simulink model "vienna"  (R2021a)
settings: Solver=VariableStepAuto  StartTime=0.0  StopTime=10.0  RelTol=1e-3
libraries: spsDiodeLib x6, spsMosfetLib x6, pid_lib x4, spsSeriesRLCBranchLib x3, spsVoltageMeasurementLib x3, powerlib_extras x3, simulink x1, spsThreePhaseSeriesRLCBranchLib x1, spsThreePhaseVIMeasurementLib x1, spsThreePhaseSourceLib x1, spsPLL3phLib x1, spspowerguiLib x1
settings Model: Creator=DSH  LastModifiedBy=DSH

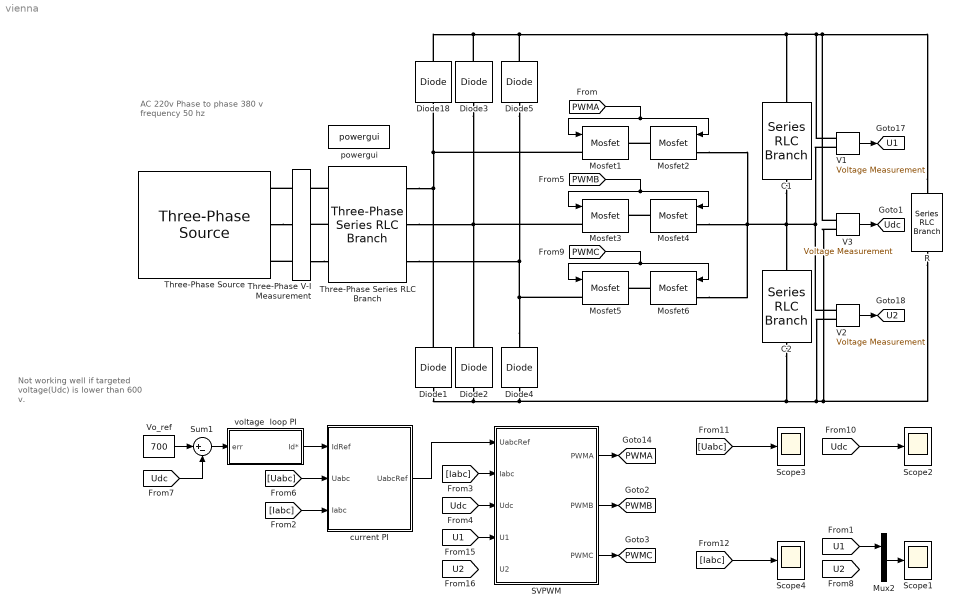
== system vienna ==
  note: AC 220v
      | Phase to phase 380 v
      | frequency 50 hz
  note: Not working well if
      | targeted voltage(Udc)
      | is lower than 600 v.
  C1 : spsSeriesRLCBranchLib/Series RLC Branch  LConnTagsString=__new0  RConnTagsString=__new0  BranchType=C  Resistance=0.1  Inductance=1e-3  SetiL0=off  InitialCurrent=0  Capacitance=1087e-6  Setx0=on  InitialVoltage=0  Measurements=None
  C2 : spsSeriesRLCBranchLib/Series RLC Branch  LConnTagsString=__new0  RConnTagsString=__new0  BranchType=C  Resistance=0.1  Inductance=1e-3  SetiL0=off  InitialCurrent=0  Capacitance=1087e-6  Setx0=on  InitialVoltage=0  Measurements=None
  Diode{1..5,18} (6 alike) : spsDiodeLib/Diode  Ron=0.001  Lon=0  Vf=0.8  IC=0  UseSnubber=off  Rs=500  Cs=250e-9  Measurements=off
  Mosfet{1..6} (6 alike) : spsMosfetLib/Mosfet  Ron=0.1  Lon=0  Rd=0.01  Vfd=0  IC=0  Rs=1e5  Cs=inf  Measurements=off
  Mux2 : Mux  Inputs=2
  R : spsSeriesRLCBranchLib/Series RLC Branch  LConnTagsString=__new0  RConnTagsString=__new0  BranchType=R  Resistance=10  Inductance=1e-3  SetiL0=off  InitialCurrent=0  Capacitance=100e-6  Setx0=off  InitialVoltage=0  Measurements=None
  SVPWM : Subsystem
  Scope{1..4} (4 alike) : Scope
  Sum1 : Sum  Inputs=|+-  SampleTime=1e-5
  Three-Phase Series RLC Branch : spsThreePhaseSeriesRLCBranchLib/Three-Phase Series RLC Branch  LConnTagsString=A|B|C  RConnTagsString=A|B|C  BranchType=L  Resistance=0.05  Inductance=0.406e-3  Capacitance=1e-6  Measurements=None
  Three-Phase V-I Measurement : spsThreePhaseVIMeasurementLib/Three-Phase V-I Measurement  VoltageMeasurement=phase-to-ground  SetLabelV=on  LabelV=Uabc  Vpu=off  VpuLL=off  CurrentMeasurement=yes  SetLabelI=on  LabelI=Iabc  Ipu=off  Pbase=100e6  Vbase=500e3  OutputType=Complex  PhasorSimulation=off  PSBequivalent=0
  Three-Phase Source : spsThreePhaseSourceLib/Three-Phase Source  InternalConnection=Yg  VoltagePhases=off  Voltage=380  PhaseAngle=0  Voltage_phases=[25e3 25e3 25e3]/sqrt(3)  PhaseAngles_phases=[0 -120 +120]  Frequency=50  NonIdealSource=on  SpecifyImpedance=off  Resistance=0.000001  Inductance=0  ShortCircuitLevel=100e6  BaseVoltage=25e3  XRratio=7  BusType=swing  Pref=0  Qref=0  Prefabc=[10e3, 10e3, 10e3]  Qrefabc=[0, 0, 0]  Qmin=-inf  Qmax=inf
  V1 : spsVoltageMeasurementLib/Voltage Measurement  PhasorSimulation=off  OutputType=Complex  PSBequivalent=0
  V2 : spsVoltageMeasurementLib/Voltage Measurement  PhasorSimulation=off  OutputType=Complex  PSBequivalent=0
  V3 : spsVoltageMeasurementLib/Voltage Measurement  PhasorSimulation=off  OutputType=Complex  PSBequivalent=0
  Vo_ref : Constant  Value=700
  current PI : Subsystem
  powergui : spspowerguiLib/powergui  Priority=1  SimulationMode=Discrete  SampleTime=1e-7  frequency=60  Iterations=50  frequencyindice=0  Pbase=100e6  ErrMax=1e-4  UnitsV=kV  UnitsW=MW  buscounter=0  FunctionMessages=off  echomessages=off  EnableUseOfTLC=off  CurrentSourceSwitches=off  DisableSnubberDevices=off  DisableRonSwitches=off  DisableVfSwitches=off  DisplayEquations=off  AutomaticDiscreteSolvers=off  SolverType=Tustin  Interpol=off  ExternalGateDelay=off  methode=off  Ts=0  x0status=blocks  SPID=off  SwTol=0  HookPort=off  NonlinearTolerance=1e-4  nMaxIteration=100  ContinueOnMaxIteration=off  RestoreLinks=warning  ResistiveCurrentMeasurement=off  Frange=[0:2:500]  Ylog=off  Xlog=on  ShowGrid=off  save=off  variable=ZData  structure=output  ZoomFFT=off  StartTime=0.1  cycles=20  DisplayStyle=1  fundamental=400  FreqAxis=off  MaxFrequency=20000  frequencyindicesteady=1  RmsSteady=1  display=off
  voltage  loop PI : Subsystem
      mask Display: disp('PI')
  tag scope: PWMA=global, PWMB=global, PWMC=global, U1=global, U2=global, Udc=global
  wires:
  [Iabc] -> Scope4/1
  [Iabc] -> SVPWM/2(Iabc)
  [Iabc] -> current PI/3(Iabc)
  Sum1/1 -> voltage  loop PI/1(err)
  [Uabc] -> Scope3/1
  [U1] -> Mux2/1
  [U1] -> SVPWM/4(U1)
  SVPWM/1(PWMA) -> [PWMA]
  Mux2/1 -> Scope1/1
  [Udc] -> Scope2/1
  V3/1 -> [Udc]
  [PWMB] -> Mosfet4/1, Mosfet3/1
  [PWMC] -> Mosfet5/1, Mosfet6/1
  [PWMA] -> Mosfet1/1, Mosfet2/1
  voltage  loop PI/1(Id*) -> current PI/1(IdRef)
  [Udc] -> SVPWM/3(Udc)
  [Uabc] -> current PI/2(Uabc)
  V2/1 -> [U2]
  Vo_ref/1 -> Sum1/1
  SVPWM/2(PWMB) -> [PWMB]
  [Udc] -> Sum1/2
  SVPWM/3(PWMC) -> [PWMC]
  V1/1 -> [U1]
  current PI/1(UabcRef) -> SVPWM/1(UabcRef)
  connections:
  R/LConn1 -- Diode5/RConn1 -- Diode18/RConn1 -- Diode3/RConn1 -- C1/LConn1 -- V1/LConn1 -- V3/LConn1
  Three-Phase Series RLC Branch/RConn1 -- Diode1/RConn1 -- Mosfet1/LConn1 -- Diode18/LConn1
  Diode4/LConn1 -- Diode1/LConn1 -- Diode2/LConn1 -- C2/RConn1 -- V2/LConn2 -- R/RConn1 -- V3/LConn2
  Three-Phase Series RLC Branch/RConn2 -- Diode3/LConn1 -- Mosfet3/LConn1 -- Diode2/RConn1
  V1/LConn2 -- Mosfet2/LConn1 -- Mosfet6/LConn1 -- Mosfet4/LConn1 -- C2/LConn1 -- C1/RConn1 -- V2/LConn1
  Diode4/RConn1 -- Diode5/LConn1 -- Three-Phase Series RLC Branch/RConn3 -- Mosfet5/LConn1
  Three-Phase Series RLC Branch/LConn1 -- Three-Phase V-I Measurement/RConn1
  Mosfet4/RConn1 -- Mosfet3/RConn1
  Mosfet6/RConn1 -- Mosfet5/RConn1
  Mosfet2/RConn1 -- Mosfet1/RConn1
  Three-Phase V-I Measurement/LConn1 -- Three-Phase Source/RConn1
  Three-Phase V-I Measurement/RConn3 -- Three-Phase Series RLC Branch/LConn3
  Three-Phase Series RLC Branch/LConn2 -- Three-Phase V-I Measurement/RConn2
  Three-Phase Source/RConn2 -- Three-Phase V-I Measurement/LConn2
  Three-Phase V-I Measurement/LConn3 -- Three-Phase Source/RConn3

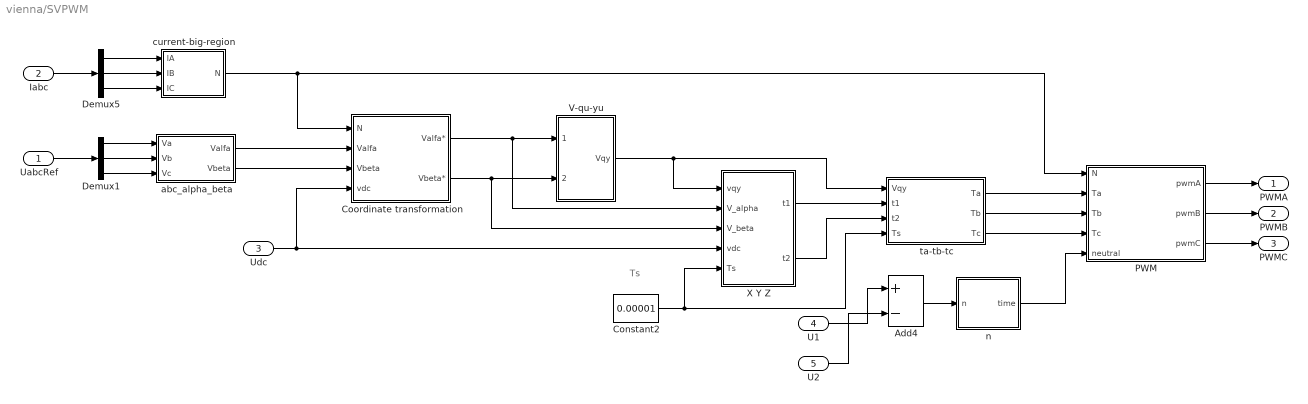
== system vienna/SVPWM ==
  note: Ts
  UabcRef : Inport
  Iabc : Inport  Port=2
  Udc : Inport  Port=3
  U1 : Inport  Port=4
  U2 : Inport  Port=5
  Add4 : Sum  Inputs=+-
  Constant2 : Constant  Value=0.00001
  Coordinate transformation : Subsystem
  Demux1 : Demux  Outputs=3
  Demux5 : Demux  Outputs=3
  PWM : Subsystem
  "V-qu-yu " : Subsystem
  X Y Z : Subsystem
  abc_alpha_beta : Subsystem
  current-big-region : Subsystem
  n : Subsystem
  ta-tb-tc : Subsystem
  PWMA : Outport
  PWMB : Outport  Port=2
  PWMC : Outport  Port=3
  wires:
  Demux1/3 -> abc_alpha_beta/3(Vc)
  Demux1/2 -> abc_alpha_beta/2(Vb)
  Demux1/1 -> abc_alpha_beta/1(Va)
  Demux5/2 -> current-big-region/2(IB)
  Demux5/1 -> current-big-region/1(IA)
  Demux5/3 -> current-big-region/3("IC ")
  abc_alpha_beta/2(Vbeta) -> Coordinate transformation/3("Vbeta ")
  Udc/1 -> X Y Z/4(vdc), Coordinate transformation/4(vdc)
  Coordinate transformation/2(Vbeta*) -> "V-qu-yu "/2(Vbeta*), X Y Z/3(V_beta)
  Coordinate transformation/1(Valfa*) -> "V-qu-yu "/1(Valfa*), X Y Z/2(V_alpha)
  Constant2/1 -> X Y Z/5(Ts), ta-tb-tc/4(Ts)
  X Y Z/1(t1) -> ta-tb-tc/2(t1)
  X Y Z/2(t2) -> ta-tb-tc/3(t2)
  ta-tb-tc/2(Tb) -> PWM/3(Tb)
  ta-tb-tc/3(Tc) -> PWM/4(Tc)
  current-big-region/1("N ") -> Coordinate transformation/1(N), PWM/1(N)
  "V-qu-yu "/1("Vqy ") -> ta-tb-tc/1(Vqy), X Y Z/1(vqy)
  ta-tb-tc/1(Ta) -> PWM/2(Ta)
  abc_alpha_beta/1(Valfa) -> Coordinate transformation/2(Valfa)
  Iabc/1 -> Demux5/1
  UabcRef/1 -> Demux1/1
  n/1(time) -> PWM/5(neutral)
  Add4/1 -> n/1(n)
  U1/1 -> Add4/1
  U2/1 -> Add4/2
  PWM/1(pwmA) -> PWMA/1
  PWM/2(pwmB) -> PWMB/1
  PWM/3(pwmC) -> PWMC/1

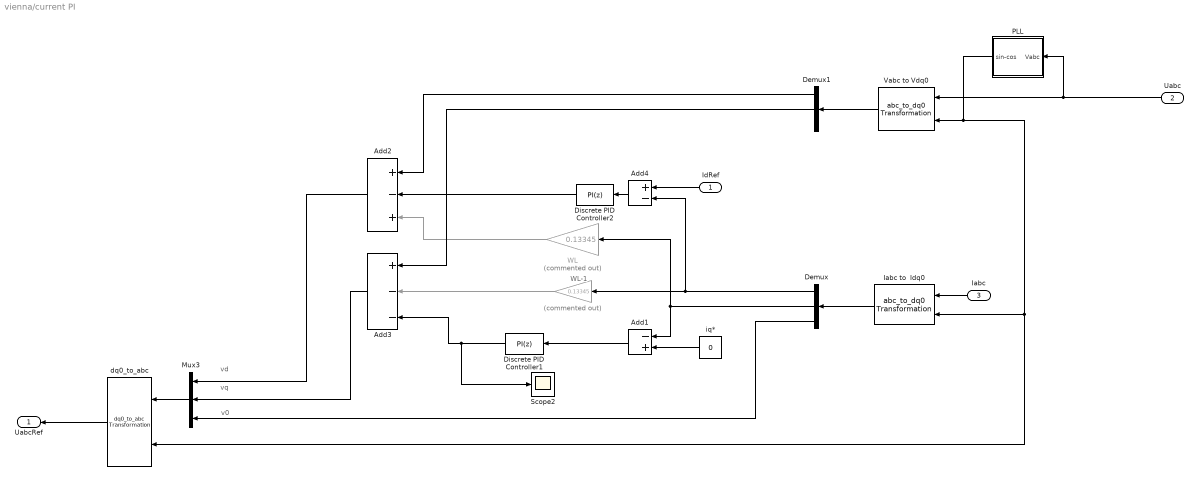
== system vienna/current PI ==
  note: v0
  note: vq
  note: vd
  note: WL-1
  IdRef : Inport
  Uabc : Inport  Port=2
  Iabc : Inport  Port=3
  " " : Gain  Commented=on  Gain=0.13345
  " WL" : Gain  Commented=on  Gain=0.13345
  Add1 : Sum  Inputs=-+
  Add2 : Sum  Inputs=+-+
  Add3 : Sum  Inputs=+--
  Add4 : Sum  Inputs=+-
  Demux : Demux  Outputs=3
  Demux1 : Demux  Outputs=3
  Discrete PID Controller1 : pid_lib/PID Controller  Controller=PI  Form=Parallel  TimeDomain=Discrete-time  UseExternalTs=off  SampleTime=1e-5  IntegratorMethod=Forward Euler  FilterMethod=Forward Euler  ControllerParametersSource=internal  P=0.1  I=100  D=0  UseFilter=on  N=100  TunerSelectOption=Transfer Function Based (PID Tuner App)  InitialConditionSource=internal  InitialConditionForIntegrator=0  InitialConditionForFilter=0  DifferentiatorICPrevScaledInput=0  ExternalReset=none  TrackingMode=off  Kt=1  LimitOutput=on  SatLimitsSource=internal  UpperSaturationLimit=600  LowerSaturationLimit=-600  LinearizeAsGain=off  AntiWindupMode=none  Kb=1  POutMin=[]  POutMax=[]  IOutMin=[]  IOutMax=[]  DOutMin=[]  DOutMax=[]  NOutMin=[]  NOutMax=[]  SumOutMin=[]  SumOutMax=[]  SaturationOutMin=[]  SaturationOutMax=[]  PParamMin=[]  PParamMax=[]  IParamMin=[]  IParamMax=[]  DParamMin=[]  DParamMax=[]  NParamMin=[]  NParamMax=[]  KbParamMin=[]  KbParamMax=[]  KtParamMin=[]  KtParamMax=[]  KbOutMin=[]  KbOutMax=[]  KtOutMin=[]  KtOutMax=[]  IntegratorOutMin=[]  IntegratorOutMax=[]  FilterOutMin=[]  FilterOutMax=[]  SumI1OutMin=[]  SumI1OutMax=[]  SumI2OutMin=[]  SumI2OutMax=[]  SumI3OutMin=[]  SumI3OutMax=[]  SumI4OutMin=[]  SumI4OutMax=[]  SumDOutMin=[]  SumDOutMax=[]  DifferentiatorOutMin=[]  DifferentiatorOutMax=[]  FilterDiffOutCoefMin=[]  FilterDiffOutCoefMax=[]  ReciprocalOutMin=[]  ReciprocalOutMax=[]  SumDenOutMin=[]  SumDenOutMax=[]  SumNumOutMin=[]  SumNumOutMax=[]  DivideOutMin=[]  DivideOutMax=[]  UdiffTsProdOutMin=[]  UdiffTsProdOutMax=[]  NTsProdOutMin=[]  NTsProdOutMax=[]  UintegralTsProdOutMin=[]  UintegralTsProdOutMax=[]  UngainTsProdOutMin=[]  UngainTsProdOutMax=[]  IntegratorContinuousStateAttributes=''  IntegratorStateMustResolveToSignalObject=off  IntegratorRTWStateStorageClass=Auto  FilterContinuousStateAttributes=''  FilterStateMustResolveToSignalObject=off  FilterRTWStateStorageClass=Auto  ParallelPVariant=InternalParameters  IdealPVariant=Disabled  IVariant=InternalParameters  DVariant=Disabled  IntegratorVariant=Discrete  SatVariant=Enabled  AWVariant=Passthrough  PCopyVariant=Disabled  TRVariant=Disabled  FdbkBlocksVariant=Forward  IdealPFdbkVariant=Disabled  SatFdbkVariant=Disabled  DerivativeFilterVariant=Disabled  NVariant=Disabled  NCopyVariant=Disabled_SignalSpec  FilterICVariant=Disabled  IntegratorICVariant=InternalICs  ExternalResetVariant=Disabled  TRSumVariant=Passthrough  SumFdbkVariant=Disabled  SumVariant=Sum_PI  TsampFilterVariant=InternalTs  TsampNgainVariant=Passthrough  TsampIntegralVariant=Passthrough  ExternalSaturationOutDataTypeStr=Inherit: Same as second input
  Discrete PID Controller2 : pid_lib/PID Controller  Controller=PI  Form=Parallel  TimeDomain=Discrete-time  UseExternalTs=off  SampleTime=1e-5  IntegratorMethod=Forward Euler  FilterMethod=Forward Euler  ControllerParametersSource=internal  P=0.1  I=100  D=0  UseFilter=on  N=100  TunerSelectOption=Transfer Function Based (PID Tuner App)  InitialConditionSource=internal  InitialConditionForIntegrator=0  InitialConditionForFilter=0  DifferentiatorICPrevScaledInput=0  ExternalReset=none  TrackingMode=off  Kt=1  LimitOutput=on  SatLimitsSource=internal  UpperSaturationLimit=600  LowerSaturationLimit=-600  LinearizeAsGain=off  AntiWindupMode=none  Kb=1  POutMin=[]  POutMax=[]  IOutMin=[]  IOutMax=[]  DOutMin=[]  DOutMax=[]  NOutMin=[]  NOutMax=[]  SumOutMin=[]  SumOutMax=[]  SaturationOutMin=[]  SaturationOutMax=[]  PParamMin=[]  PParamMax=[]  IParamMin=[]  IParamMax=[]  DParamMin=[]  DParamMax=[]  NParamMin=[]  NParamMax=[]  KbParamMin=[]  KbParamMax=[]  KtParamMin=[]  KtParamMax=[]  KbOutMin=[]  KbOutMax=[]  KtOutMin=[]  KtOutMax=[]  IntegratorOutMin=[]  IntegratorOutMax=[]  FilterOutMin=[]  FilterOutMax=[]  SumI1OutMin=[]  SumI1OutMax=[]  SumI2OutMin=[]  SumI2OutMax=[]  SumI3OutMin=[]  SumI3OutMax=[]  SumI4OutMin=[]  SumI4OutMax=[]  SumDOutMin=[]  SumDOutMax=[]  DifferentiatorOutMin=[]  DifferentiatorOutMax=[]  FilterDiffOutCoefMin=[]  FilterDiffOutCoefMax=[]  ReciprocalOutMin=[]  ReciprocalOutMax=[]  SumDenOutMin=[]  SumDenOutMax=[]  SumNumOutMin=[]  SumNumOutMax=[]  DivideOutMin=[]  DivideOutMax=[]  UdiffTsProdOutMin=[]  UdiffTsProdOutMax=[]  NTsProdOutMin=[]  NTsProdOutMax=[]  UintegralTsProdOutMin=[]  UintegralTsProdOutMax=[]  UngainTsProdOutMin=[]  UngainTsProdOutMax=[]  IntegratorContinuousStateAttributes=''  IntegratorStateMustResolveToSignalObject=off  IntegratorRTWStateStorageClass=Auto  FilterContinuousStateAttributes=''  FilterStateMustResolveToSignalObject=off  FilterRTWStateStorageClass=Auto  ParallelPVariant=InternalParameters  IdealPVariant=Disabled  IVariant=InternalParameters  DVariant=Disabled  IntegratorVariant=Discrete  SatVariant=Enabled  AWVariant=Passthrough  PCopyVariant=Disabled  TRVariant=Disabled  FdbkBlocksVariant=Forward  IdealPFdbkVariant=Disabled  SatFdbkVariant=Disabled  DerivativeFilterVariant=Disabled  NVariant=Disabled  NCopyVariant=Disabled_SignalSpec  FilterICVariant=Disabled  IntegratorICVariant=InternalICs  ExternalResetVariant=Disabled  TRSumVariant=Passthrough  SumFdbkVariant=Disabled  SumVariant=Sum_PI  TsampFilterVariant=InternalTs  TsampNgainVariant=Passthrough  TsampIntegralVariant=Passthrough  ExternalSaturationOutDataTypeStr=Inherit: Same as second input
  Iabc to  Idq0 : powerlib_extras/Measurements/abc_to_dq0 Transformation
      settings: SourceProductBaseCode=PS
  Mux3 : Mux  Inputs=3
  PLL : Subsystem
  Scope2 : Scope
  Vabc to Vdq0 : powerlib_extras/Measurements/abc_to_dq0 Transformation
      settings: SourceProductBaseCode=PS
  dq0_to_abc : powerlib_extras/Measurements/dq0_to_abc Transformation
      settings: SourceProductBaseCode=PS
  iq* : Constant  Value=0
  UabcRef : Outport
  wires:
  " WL"/1 -> Add2/3
  Discrete PID Controller2/1 -> Add2/2
  Demux1/1 -> Add2/1
  Vabc to Vdq0/1 -> Demux1/1
  Uabc/1 -> Vabc to Vdq0/1, PLL/1(Vabc)
  Add3/1 -> Mux3/2
  Add2/1 -> Mux3/1
  Mux3/1 -> dq0_to_abc/1
  Demux/1 -> Add4/2, " "/1
  Demux/3 -> Mux3/3
  dq0_to_abc/1 -> UabcRef/1
  Iabc/1 -> Iabc to  Idq0/1
  Add1/1 -> Discrete PID Controller1/1
  Iabc to  Idq0/1 -> Demux/1
  IdRef/1 -> Add4/1
  Discrete PID Controller1/1 -> Scope2/1, Add3/3
  Demux1/2 -> Add3/1
  " "/1 -> Add3/2
  PLL/1(sin-cos) -> Vabc to Vdq0/2, dq0_to_abc/2, Iabc to  Idq0/2
  Demux/2 -> " WL"/1, Add1/1
  iq*/1 -> Add1/2
  Add4/1 -> Discrete PID Controller2/1

== system vienna/voltage  loop PI ==
  err : Inport
  Discrete PID Controller : pid_lib/PID Controller  Controller=PI  Form=Parallel  TimeDomain=Discrete-time  UseExternalTs=off  SampleTime=1e-5  IntegratorMethod=Forward Euler  FilterMethod=Forward Euler  ControllerParametersSource=internal  P=0.5  I=100  D=0  UseFilter=on  N=100  TunerSelectOption=Transfer Function Based (PID Tuner App)  InitialConditionSource=internal  InitialConditionForIntegrator=0  InitialConditionForFilter=0  DifferentiatorICPrevScaledInput=0  ExternalReset=none  TrackingMode=off  Kt=1  LimitOutput=on  SatLimitsSource=internal  UpperSaturationLimit=150  LowerSaturationLimit=0  LinearizeAsGain=off  AntiWindupMode=none  Kb=1  POutMin=[]  POutMax=[]  IOutMin=[]  IOutMax=[]  DOutMin=[]  DOutMax=[]  NOutMin=[]  NOutMax=[]  SumOutMin=[]  SumOutMax=[]  SaturationOutMin=[]  SaturationOutMax=[]  PParamMin=[]  PParamMax=[]  IParamMin=[]  IParamMax=[]  DParamMin=[]  DParamMax=[]  NParamMin=[]  NParamMax=[]  KbParamMin=[]  KbParamMax=[]  KtParamMin=[]  KtParamMax=[]  KbOutMin=[]  KbOutMax=[]  KtOutMin=[]  KtOutMax=[]  IntegratorOutMin=[]  IntegratorOutMax=[]  FilterOutMin=[]  FilterOutMax=[]  SumI1OutMin=[]  SumI1OutMax=[]  SumI2OutMin=[]  SumI2OutMax=[]  SumI3OutMin=[]  SumI3OutMax=[]  SumI4OutMin=[]  SumI4OutMax=[]  SumDOutMin=[]  SumDOutMax=[]  DifferentiatorOutMin=[]  DifferentiatorOutMax=[]  FilterDiffOutCoefMin=[]  FilterDiffOutCoefMax=[]  ReciprocalOutMin=[]  ReciprocalOutMax=[]  SumDenOutMin=[]  SumDenOutMax=[]  SumNumOutMin=[]  SumNumOutMax=[]  DivideOutMin=[]  DivideOutMax=[]  UdiffTsProdOutMin=[]  UdiffTsProdOutMax=[]  NTsProdOutMin=[]  NTsProdOutMax=[]  UintegralTsProdOutMin=[]  UintegralTsProdOutMax=[]  UngainTsProdOutMin=[]  UngainTsProdOutMax=[]  IntegratorContinuousStateAttributes=''  IntegratorStateMustResolveToSignalObject=off  IntegratorRTWStateStorageClass=Auto  FilterContinuousStateAttributes=''  FilterStateMustResolveToSignalObject=off  FilterRTWStateStorageClass=Auto  ParallelPVariant=InternalParameters  IdealPVariant=Disabled  IVariant=InternalParameters  DVariant=Disabled  IntegratorVariant=Discrete  SatVariant=Enabled  AWVariant=Passthrough  PCopyVariant=Disabled  TRVariant=Disabled  FdbkBlocksVariant=Forward  IdealPFdbkVariant=Disabled  SatFdbkVariant=Disabled  DerivativeFilterVariant=Disabled  NVariant=Disabled  NCopyVariant=Disabled_SignalSpec  FilterICVariant=Disabled  IntegratorICVariant=InternalICs  ExternalResetVariant=Disabled  TRSumVariant=Passthrough  SumFdbkVariant=Disabled  SumVariant=Sum_PI  TsampFilterVariant=InternalTs  TsampNgainVariant=Passthrough  TsampIntegralVariant=Passthrough  ExternalSaturationOutDataTypeStr=Inherit: Same as second input
  Id* : Outport
  wires:
  err/1 -> Discrete PID Controller/1
  Discrete PID Controller/1 -> Id*/1

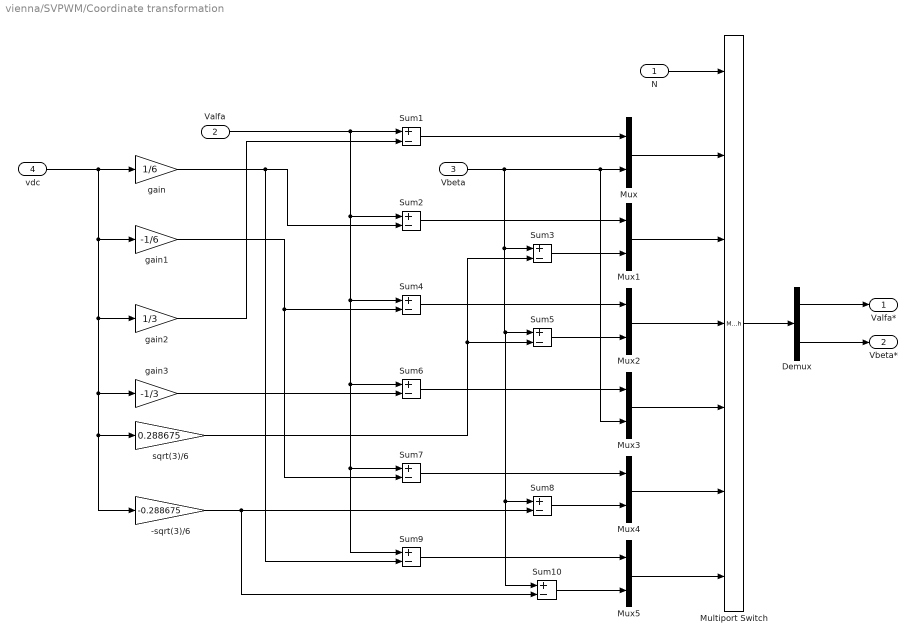
== system vienna/SVPWM/Coordinate transformation ==
  N : Inport
  Valfa : Inport  Port=2
  "Vbeta " : Inport  Port=3
  vdc : Inport  Port=4
  -sqrt(3)/6 : Gain  Gain=-0.288675
  Demux : Demux  Outputs=2
  Multiport Switch : MultiPortSwitch  Inputs=6
  Mux{,1..5} (6 alike) : Mux  Inputs=2
  Sum{1..10} (10 alike) : Sum  Inputs=+-  SaturateOnIntegerOverflow=on
  gain : Gain  Gain=1/6
  gain1 : Gain  Gain=-1/6
  gain2 : Gain  Gain=1/3
  gain3 : Gain  Gain=-1/3
  sqrt(3)/6 : Gain  Gain=0.288675
  Valfa* : Outport
  Vbeta* : Outport  Port=2
  wires:
  Multiport Switch/1 -> Demux/1
  Demux/1 -> Valfa*/1
  Demux/2 -> Vbeta*/1
  N/1 -> Multiport Switch/1
  Mux/1 -> Multiport Switch/2
  Mux1/1 -> Multiport Switch/3
  Mux2/1 -> Multiport Switch/4
  Mux3/1 -> Multiport Switch/5
  Mux4/1 -> Multiport Switch/6
  Mux5/1 -> Multiport Switch/7
  vdc/1 -> gain/1, gain1/1, gain2/1, gain3/1, sqrt(3)/6/1, -sqrt(3)/6/1
  gain2/1 -> Sum1/2
  Valfa/1 -> Sum1/1, Sum6/1, Sum7/1, Sum9/1, Sum4/1, Sum2/1
  Sum1/1 -> Mux/1
  "Vbeta "/1 -> Sum10/1, Sum8/1, Sum5/1, Sum3/1, Mux3/2, Mux/2
  Sum2/1 -> Mux1/1
  Sum3/1 -> Mux1/2
  Sum4/1 -> Mux2/1
  Sum5/1 -> Mux2/2
  Sum6/1 -> Mux3/1
  Sum7/1 -> Mux4/1
  Sum8/1 -> Mux4/2
  Sum9/1 -> Mux5/1
  Sum10/1 -> Mux5/2
  gain/1 -> Sum9/2, Sum2/2
  gain1/1 -> Sum7/2, Sum4/2
  gain3/1 -> Sum6/2
  sqrt(3)/6/1 -> Sum5/2, Sum3/2
  -sqrt(3)/6/1 -> Sum8/2, Sum10/2

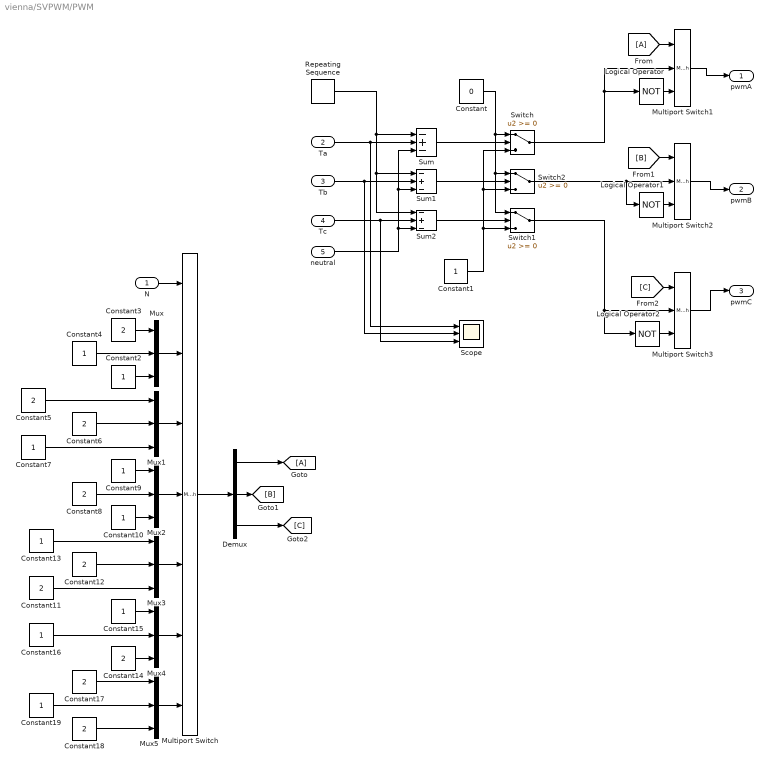
== system vienna/SVPWM/PWM ==
  N : Inport
  Ta : Inport  Port=2
  Tb : Inport  Port=3
  Tc : Inport  Port=4
  neutral : Inport  Port=5
  Constant : Constant  Value=0
  Constant{1..2,4,7,9..10,13,15..16,19} (10 alike) : Constant
  Constant{3,5..6,8,11..12,14,17..18} (9 alike) : Constant  Value=2
  Demux : Demux  Outputs=3
  Logical Operator : Logic  Operator=NOT  AllPortsSameDT=off  OutDataTypeStr=boolean
  Logical Operator1 : Logic  Operator=NOT  AllPortsSameDT=off  OutDataTypeStr=boolean
  Logical Operator2 : Logic  Operator=NOT  AllPortsSameDT=off  OutDataTypeStr=boolean
  Multiport Switch : MultiPortSwitch  Inputs=6
  Multiport Switch1 : MultiPortSwitch  Inputs=2
  Multiport Switch2 : MultiPortSwitch  Inputs=2
  Multiport Switch3 : MultiPortSwitch  Inputs=2
  Mux{,1..5} (6 alike) : Mux  Inputs=3
  Repeating Sequence : simulink/Sources/Repeating Sequence  rep_seq_t=[0 0.000005 0.00001]  rep_seq_y=[0 0.000005 0]
  Scope : Scope  NumInputPorts=3
  Sum : Sum  Inputs=-+-  SaturateOnIntegerOverflow=on
  Sum1 : Sum  Inputs=-+-  SaturateOnIntegerOverflow=on
  Sum2 : Sum  Inputs=-+-  SaturateOnIntegerOverflow=on
  Switch : Switch  SaturateOnIntegerOverflow=on
  Switch1 : Switch  SaturateOnIntegerOverflow=on
  Switch2 : Switch  SaturateOnIntegerOverflow=on
  pwmA : Outport
  pwmB : Outport  Port=2
  pwmC : Outport  Port=3
  wires:
  Sum2/1 -> Switch1/2
  Sum1/1 -> Switch2/2
  Constant/1 -> Switch/1, Switch2/1, Switch1/1
  Constant1/1 -> Switch1/3, Switch2/3, Switch/3
  Sum/1 -> Switch/2
  Repeating Sequence/1 -> Sum2/1, Sum1/1, Sum/1
  N/1 -> Multiport Switch/1
  Switch/1 -> Logical Operator/1, Multiport Switch1/2
  Switch2/1 -> Logical Operator1/1, Multiport Switch2/2
  Switch1/1 -> Multiport Switch3/2, Logical Operator2/1
  Logical Operator/1 -> Multiport Switch1/3
  Logical Operator1/1 -> Multiport Switch2/3
  Logical Operator2/1 -> Multiport Switch3/3
  Multiport Switch/1 -> Demux/1
  Demux/1 -> [A]
  Demux/2 -> [B]
  Demux/3 -> [C]
  [A] -> Multiport Switch1/1
  [B] -> Multiport Switch2/1
  [C] -> Multiport Switch3/1
  Mux/1 -> Multiport Switch/2
  Mux1/1 -> Multiport Switch/3
  Mux2/1 -> Multiport Switch/4
  Mux3/1 -> Multiport Switch/5
  Mux4/1 -> Multiport Switch/6
  Mux5/1 -> Multiport Switch/7
  Constant5/1 -> Mux1/1
  Constant7/1 -> Mux1/3
  Constant9/1 -> Mux2/1
  Constant10/1 -> Mux2/3
  Constant11/1 -> Mux3/3
  Constant13/1 -> Mux3/1
  Constant14/1 -> Mux4/3
  Constant15/1 -> Mux4/1
  Constant17/1 -> Mux5/1
  Constant18/1 -> Mux5/3
  Constant3/1 -> Mux/1
  Constant4/1 -> Mux/2
  Constant2/1 -> Mux/3
  Constant6/1 -> Mux1/2
  Constant8/1 -> Mux2/2
  Constant12/1 -> Mux3/2
  Constant16/1 -> Mux4/2
  Constant19/1 -> Mux5/2
  Ta/1 -> Scope/1, Sum/2
  Tb/1 -> Scope/2, Sum1/2
  ? -> ?
  Tc/1 -> Scope/3, Sum2/2
  neutral/1 -> Sum2/3, Sum1/3, Sum/3
  Multiport Switch1/1 -> pwmA/1
  Multiport Switch2/1 -> pwmB/1
  Multiport Switch3/1 -> pwmC/1

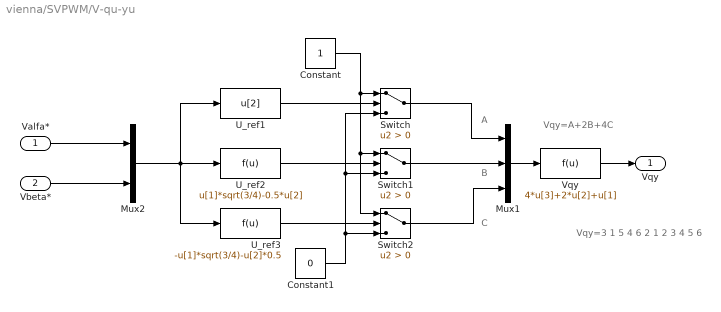
== system vienna/SVPWM/V-qu-yu  ==
  note: A
  note: B
  note: C
  note: Vqy=A+2B+4C
  note: Vqy=3    1    5    4    6    2
      |
      |         1    2    3    4    5    6
  Valfa* : Inport
  Vbeta* : Inport  Port=2
  Constant : Constant
  Constant1 : Constant  Value=0
  Mux1 : Mux  Inputs=3
  Mux2 : Mux  Inputs=2
  Switch : Switch  Criteria=u2 > Threshold
  Switch1 : Switch  Criteria=u2 > Threshold
  Switch2 : Switch  Criteria=u2 > Threshold
  U_ref1 : Fcn  Expr=u[2]
  U_ref2 : Fcn  Expr=u[1]*sqrt(3/4)-0.5*u[2]
  U_ref3 : Fcn  Expr=-u[1]*sqrt(3/4)-u[2]*0.5
  Vqy : Fcn  Expr=4*u[3]+2*u[2]+u[1]
  "Vqy " : Outport
  wires:
  Switch2/1 -> Mux1/3
  Switch/1 -> Mux1/1
  Valfa*/1 -> Mux2/1
  Vbeta*/1 -> Mux2/2
  Mux2/1 -> U_ref2/1, U_ref1/1, U_ref3/1
  U_ref1/1 -> Switch/2
  U_ref2/1 -> Switch1/2
  U_ref3/1 -> Switch2/2
  Constant/1 -> Switch/1, Switch2/1, Switch1/1
  Constant1/1 -> Switch/3, Switch1/3, Switch2/3
  Switch1/1 -> Mux1/2
  Mux1/1 -> Vqy/1
  Vqy/1 -> "Vqy "/1

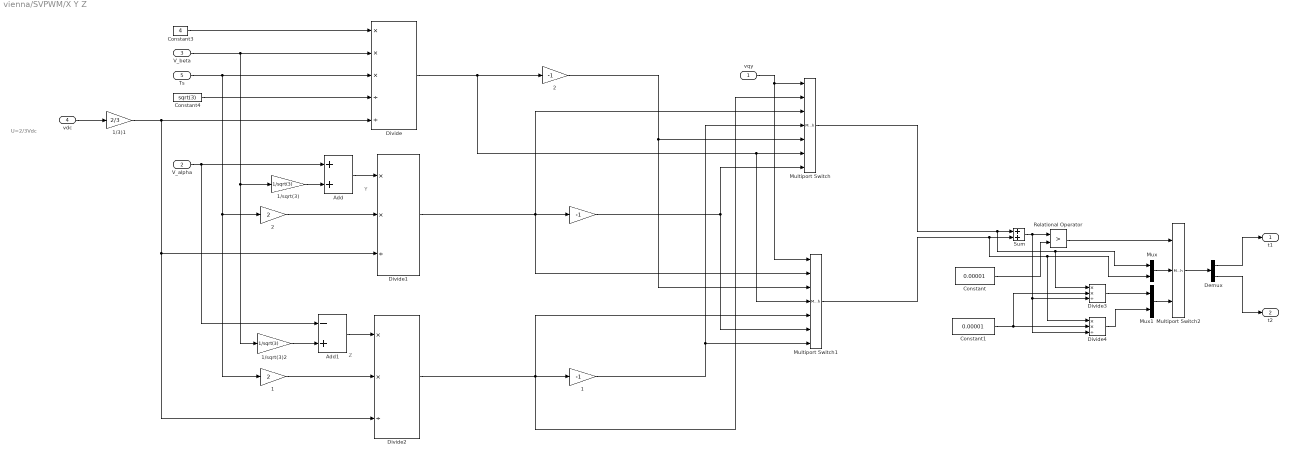
== system vienna/SVPWM/X Y Z ==
  note: U=2/3Vdc
  note: Y
  note: Z
  vqy : Inport
  V_alpha : Inport  Port=2
  V_beta : Inport  Port=3
  vdc : Inport  Port=4
  Ts : Inport  Port=5
  " " : Gain  Gain=-1
  " 1" : Gain  Gain=-1
  " 2" : Gain  Gain=-1
  1 : Gain  Gain=2
  1/3)1 : Gain  Gain=2/3
  1/sqrt(3) : Gain  Gain=1/sqrt(3)
  1/sqrt(3)2 : Gain  Gain=1/sqrt(3)
  2 : Gain  Gain=2
  Add : Sum
  Add1 : Sum  Inputs=-+
  Constant : Constant  Value=0.00001
  Constant1 : Constant  Value=0.00001
  Constant3 : Constant  Value=4
  Constant4 : Constant  Value=sqrt(3)
  Demux : Demux  Outputs=2
  Divide : Product  Inputs=***//
  Divide{1..4} (4 alike) : Product  Inputs=**/
  Multiport Switch : MultiPortSwitch  Inputs=6
  Multiport Switch1 : MultiPortSwitch  Inputs=6
  Multiport Switch2 : MultiPortSwitch  DataPortOrder=Zero-based contiguous  Inputs=2  zeroidx=on
  Mux : Mux  Inputs=2
  Mux1 : Mux  Inputs=2
  Relational Operator : RelationalOperator  Operator=>  OutDataTypeStr=boolean  RndMeth=Nearest
  Sum : Sum  SaturateOnIntegerOverflow=on
  t1 : Outport
  t2 : Outport  Port=2
  wires:
  Ts/1 -> Divide/3, 2/1, 1/1
  Constant4/1 -> Divide/4
  V_beta/1 -> Divide/2, 1/sqrt(3)/1, 1/sqrt(3)2/1
  V_alpha/1 -> Add/1, Add1/1
  1/sqrt(3)/1 -> Add/2
  Add/1 -> Divide1/1
  2/1 -> Divide1/2
  Divide1/1 -> Multiport Switch1/2, Multiport Switch/3, " "/1
  1/sqrt(3)2/1 -> Add1/2
  Add1/1 -> Divide2/1
  1/1 -> Divide2/2
  Divide2/1 -> Multiport Switch/2, Multiport Switch1/5, " 1"/1
  vqy/1 -> Multiport Switch/1, Multiport Switch1/1
  Divide/1 -> Multiport Switch/6, Multiport Switch1/4, " 2"/1
  Constant3/1 -> Divide/1
  vdc/1 -> 1/3)1/1
  1/3)1/1 -> Divide1/3, Divide2/3, Divide/5
  Multiport Switch1/1 -> Mux/2, Divide4/1, Sum/2
  Multiport Switch/1 -> Divide3/1, Mux/1, Sum/1
  Sum/1 -> Divide4/3, Divide3/3, Relational Operator/1
  Constant/1 -> Relational Operator/2
  Relational Operator/1 -> Multiport Switch2/1
  Multiport Switch2/1 -> Demux/1
  Demux/2 -> t2/1
  Demux/1 -> t1/1
  Mux/1 -> Multiport Switch2/2
  Mux1/1 -> Multiport Switch2/3
  Divide4/1 -> Mux1/2
  Divide3/1 -> Mux1/1
  Constant1/1 -> Divide3/2, Divide4/2
  " 2"/1 -> Multiport Switch/5, Multiport Switch1/3
  " 1"/1 -> Multiport Switch/4, Multiport Switch1/7
  " "/1 -> Multiport Switch/7, Multiport Switch1/6

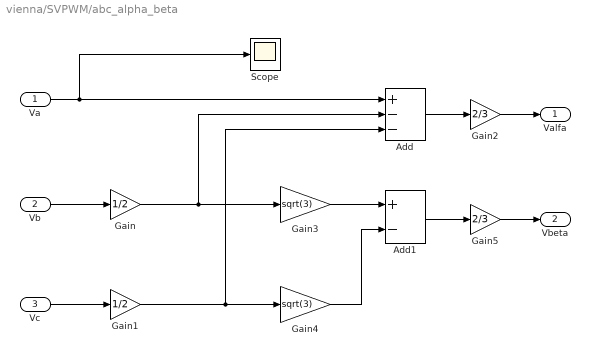
== system vienna/SVPWM/abc_alpha_beta ==
  Va : Inport
  Vb : Inport  Port=2
  Vc : Inport  Port=3
  Add : Sum  Inputs=+--
  Add1 : Sum  Inputs=+-
  Gain : Gain  Gain=1/2
  Gain1 : Gain  Gain=1/2
  Gain2 : Gain  Gain=2/3
  Gain3 : Gain  Gain=sqrt(3)
  Gain4 : Gain  Gain=sqrt(3)
  Gain5 : Gain  Gain=2/3
  Scope : Scope
  Valfa : Outport
  Vbeta : Outport  Port=2
  wires:
  Vc/1 -> Gain1/1
  Vb/1 -> Gain/1
  Va/1 -> Scope/1, Add/1
  Gain/1 -> Gain3/1, Add/2
  Gain1/1 -> Add/3, Gain4/1
  Gain3/1 -> Add1/1
  Gain4/1 -> Add1/2
  Gain2/1 -> Valfa/1
  Add/1 -> Gain2/1
  Add1/1 -> Gain5/1
  Gain5/1 -> Vbeta/1

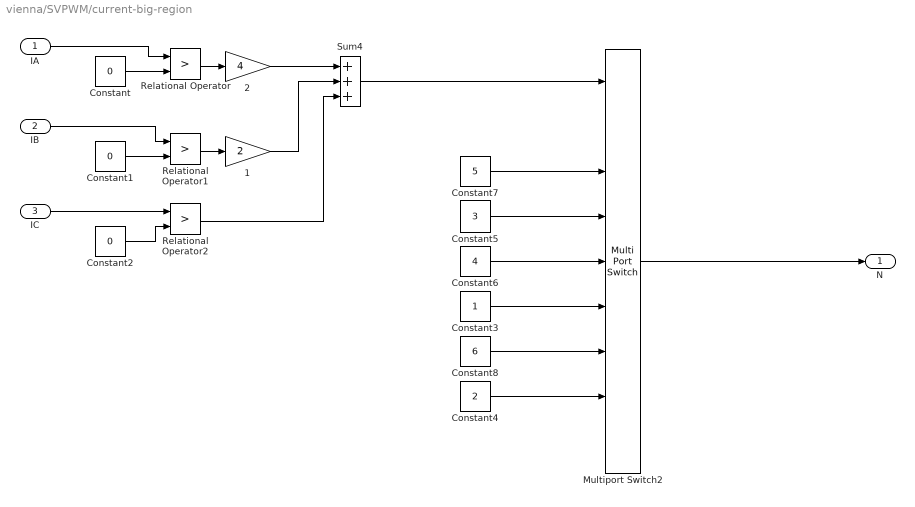
== system vienna/SVPWM/current-big-region ==
  IA : Inport
  IB : Inport  Port=2
  "IC " : Inport  Port=3
  1 : Gain  Gain=2
  2 : Gain  Gain=4
  Constant : Constant  Value=0
  Constant1 : Constant  Value=0
  Constant2 : Constant  Value=0
  Constant3 : Constant
  Constant4 : Constant  Value=2
  Constant5 : Constant  Value=3
  Constant6 : Constant  Value=4
  Constant7 : Constant  Value=5
  Constant8 : Constant  Value=6
  Multiport Switch2 : MultiPortSwitch  DataPortOrder=Zero-based contiguous  Inputs=8  zeroidx=on
  Relational Operator : RelationalOperator  Operator=>  OutDataTypeStr=boolean  ZeroCross=off  RndMeth=Nearest
  Relational Operator1 : RelationalOperator  Operator=>  OutDataTypeStr=boolean  ZeroCross=off  RndMeth=Nearest
  Relational Operator2 : RelationalOperator  Operator=>  OutDataTypeStr=boolean  ZeroCross=off  RndMeth=Nearest
  Sum4 : Sum  Inputs=+++  SaturateOnIntegerOverflow=on
  "N " : Outport
  wires:
  Constant/1 -> Relational Operator/2
  Constant1/1 -> Relational Operator1/2
  Constant2/1 -> Relational Operator2/2
  IA/1 -> Relational Operator/1
  IB/1 -> Relational Operator1/1
  "IC "/1 -> Relational Operator2/1
  Constant3/1 -> Multiport Switch2/6
  Constant4/1 -> Multiport Switch2/8
  Constant5/1 -> Multiport Switch2/4
  Constant6/1 -> Multiport Switch2/5
  Constant7/1 -> Multiport Switch2/3
  Constant8/1 -> Multiport Switch2/7
  Relational Operator/1 -> 2/1
  Relational Operator1/1 -> 1/1
  2/1 -> Sum4/1
  1/1 -> Sum4/2
  Relational Operator2/1 -> Sum4/3
  Sum4/1 -> Multiport Switch2/1
  Multiport Switch2/1 -> "N "/1

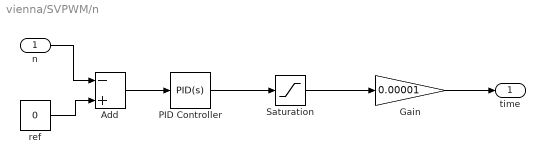
== system vienna/SVPWM/n ==
  n : Inport
  Add : Sum  Inputs=-+
  Gain : Gain  Gain=0.00001
  PID Controller : pid_lib/PID Controller  Controller=PID  Form=Parallel  TimeDomain=Continuous-time  UseExternalTs=off  SampleTime=-1  IntegratorMethod=Forward Euler  FilterMethod=Forward Euler  ControllerParametersSource=internal  P=0.2  I=1  D=0  UseFilter=on  N=100  TunerSelectOption=Transfer Function Based (PID Tuner App)  InitialConditionSource=internal  InitialConditionForIntegrator=0  InitialConditionForFilter=0  DifferentiatorICPrevScaledInput=0  ExternalReset=none  TrackingMode=off  Kt=1  LimitOutput=off  SatLimitsSource=internal  UpperSaturationLimit=inf  LowerSaturationLimit=-inf  LinearizeAsGain=on  AntiWindupMode=none  Kb=1  POutMin=[]  POutMax=[]  IOutMin=[]  IOutMax=[]  DOutMin=[]  DOutMax=[]  NOutMin=[]  NOutMax=[]  SumOutMin=[]  SumOutMax=[]  SaturationOutMin=[]  SaturationOutMax=[]  PParamMin=[]  PParamMax=[]  IParamMin=[]  IParamMax=[]  DParamMin=[]  DParamMax=[]  NParamMin=[]  NParamMax=[]  KbParamMin=[]  KbParamMax=[]  KtParamMin=[]  KtParamMax=[]  KbOutMin=[]  KbOutMax=[]  KtOutMin=[]  KtOutMax=[]  IntegratorOutMin=[]  IntegratorOutMax=[]  FilterOutMin=[]  FilterOutMax=[]  SumI1OutMin=[]  SumI1OutMax=[]  SumI2OutMin=[]  SumI2OutMax=[]  SumI3OutMin=[]  SumI3OutMax=[]  SumI4OutMin=[]  SumI4OutMax=[]  SumDOutMin=[]  SumDOutMax=[]  DifferentiatorOutMin=[]  DifferentiatorOutMax=[]  FilterDiffOutCoefMin=[]  FilterDiffOutCoefMax=[]  ReciprocalOutMin=[]  ReciprocalOutMax=[]  SumDenOutMin=[]  SumDenOutMax=[]  SumNumOutMin=[]  SumNumOutMax=[]  DivideOutMin=[]  DivideOutMax=[]  UdiffTsProdOutMin=[]  UdiffTsProdOutMax=[]  NTsProdOutMin=[]  NTsProdOutMax=[]  UintegralTsProdOutMin=[]  UintegralTsProdOutMax=[]  UngainTsProdOutMin=[]  UngainTsProdOutMax=[]  IntegratorContinuousStateAttributes=''  IntegratorStateMustResolveToSignalObject=off  IntegratorRTWStateStorageClass=Auto  FilterContinuousStateAttributes=''  FilterStateMustResolveToSignalObject=off  FilterRTWStateStorageClass=Auto  ParallelPVariant=InternalParameters  IdealPVariant=Disabled  IVariant=InternalParameters  DVariant=InternalParameters  IntegratorVariant=Continuous  SatVariant=Disabled  AWVariant=Passthrough  PCopyVariant=Disabled  TRVariant=Disabled  FdbkBlocksVariant=Forward  IdealPFdbkVariant=Disabled  SatFdbkVariant=Disabled  DerivativeFilterVariant=ContFilter  NVariant=InternalParameters  NCopyVariant=Disabled  FilterICVariant=InternalICsFilter  IntegratorICVariant=InternalICs  ExternalResetVariant=Disabled  TRSumVariant=Passthrough  SumFdbkVariant=Disabled  SumVariant=Sum_PID  TsampFilterVariant=InternalTs  TsampNgainVariant=Passthrough  TsampIntegralVariant=Passthrough  ExternalSaturationOutDataTypeStr=Inherit: Same as second input
  Saturation : Saturate  UpperLimit=1  LowerLimit=-1
  ref : Constant  Value=0
  time : Outport
  wires:
  n/1 -> Add/1
  ref/1 -> Add/2
  Add/1 -> PID Controller/1
  Saturation/1 -> Gain/1
  PID Controller/1 -> Saturation/1
  Gain/1 -> time/1

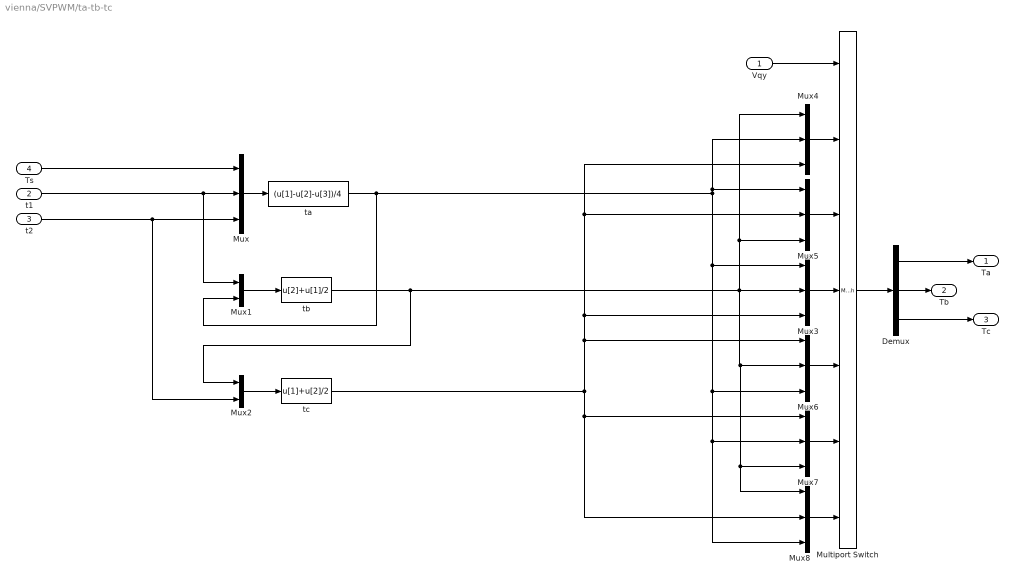
== system vienna/SVPWM/ta-tb-tc ==
  Vqy : Inport
  t1 : Inport  Port=2
  t2 : Inport  Port=3
  Ts : Inport  Port=4
  Demux : Demux  Outputs=3
  Multiport Switch : MultiPortSwitch  Inputs=6
  Mux{,3..8} (7 alike) : Mux  Inputs=3
  Mux1 : Mux  Inputs=2
  Mux2 : Mux  Inputs=2
  ta : Fcn  Expr=(u[1]-u[2]-u[3])/4
  tb : Fcn  Expr=u[2]+u[1]/2
  tc : Fcn  Expr=u[1]+u[2]/2
  Ta : Outport
  Tb : Outport  Port=2
  Tc : Outport  Port=3
  wires:
  tb/1 -> Mux4/1, Mux5/3, Mux7/3, Mux8/1, Mux6/2, Mux3/2, Mux2/1
  Ts/1 -> Mux/1
  t1/1 -> Mux1/1, Mux/2
  Mux1/1 -> tb/1
  Mux/1 -> ta/1
  Mux2/1 -> tc/1
  t2/1 -> Mux2/2, Mux/3
  ta/1 -> Mux6/3, Mux7/2, Mux8/3, Mux3/1, Mux4/2, Mux5/1, Mux1/2
  tc/1 -> Mux4/3, Mux5/2, Mux3/3, Mux6/1, Mux7/1, Mux8/2
  Vqy/1 -> Multiport Switch/1
  Multiport Switch/1 -> Demux/1
  Mux3/1 -> Multiport Switch/4
  Demux/1 -> Ta/1
  Demux/2 -> Tb/1
  Demux/3 -> Tc/1
  Mux4/1 -> Multiport Switch/2
  Mux5/1 -> Multiport Switch/3
  Mux6/1 -> Multiport Switch/5
  Mux7/1 -> Multiport Switch/6
  Mux8/1 -> Multiport Switch/7

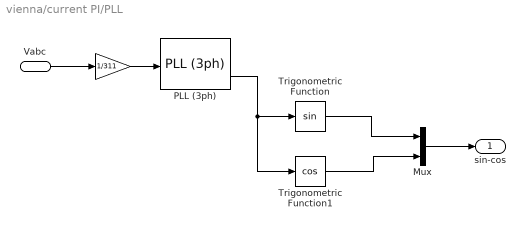
== system vienna/current PI/PLL ==
  Vabc : Inport
  " " : Gain  Gain=1/311
  Mux : Mux  Inputs=2
  PLL (3ph) : spsPLL3phLib/PLL (3ph)  Fmin=45  Par_Init=[0, 50]  ParK=[180, 3200, 1]  TcD=1e-4  MaxRateChangeFreq=12  FilterCutOffFreq=25  Ts=1e-5  AGC=on
  Trigonometric Function : Trigonometry
  Trigonometric Function1 : Trigonometry  Operator=cos
  sin-cos : Outport
  wires:
  Mux/1 -> sin-cos/1
  " "/1 -> PLL (3ph)/1
  Trigonometric Function/1 -> Mux/1
  Trigonometric Function1/1 -> Mux/2
  PLL (3ph)/2 -> Trigonometric Function1/1, Trigonometric Function/1
  Vabc/1 -> " "/1
